simulink model "GaNFET_IMMD_Thermal_Model"  (R2017a)
settings: Solver=VariableStepAuto  StartTime=0.0  StopTime=10.0  RelTol=1e-3
values from neighbouring files (symbols this model uses):
  Rth_jc_FWD2U = 0.12    [Power_loss_calculation.m]
  Rth_jc_IGBT2U = 0.066    [Power_loss_calculation.m]
libraries: fl_lib x29, nesl_utility x2
settings Model: Creator=Caner  LastModifiedBy=Caner

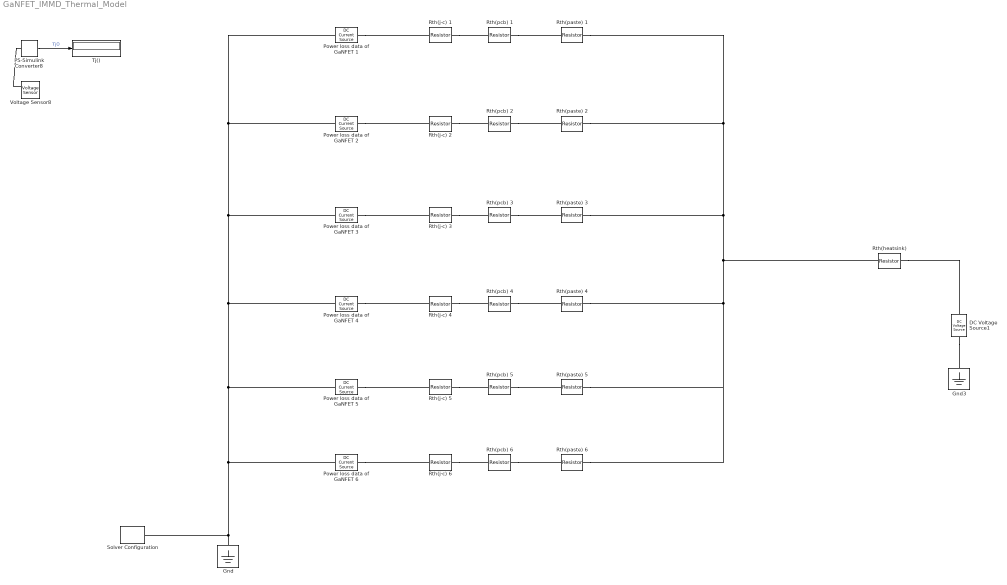
== system GaNFET_IMMD_Thermal_Model ==
  DC Voltage Source1 : fl_lib/Electrical/Electrical Sources/DC Voltage Source  v0=40 V
  Gnd : fl_lib/Electrical/Electrical Elements/Electrical Reference
  Gnd3 : fl_lib/Electrical/Electrical Elements/Electrical Reference
  PS-Simulink Converter8 : nesl_utility/PS-Simulink Converter  PhysicalDomain=network_engine_domain  SubClassName=ps_output  LeftPortType=input  RightPortType=output  PseudoPeriodic=off  Frequencies=[]  Unit=1  AffineConversion=off
  Power loss data of GaNFET 1 : fl_lib/Electrical/Electrical Sources/DC Current Source  i0=PD A
      settings: SourceProductName=Simscape  SourceProductBaseCode=SS
  Power loss data of GaNFET {2..6} (5 alike) : fl_lib/Electrical/Electrical Sources/DC Current Source  i0=PQ A
      settings: SourceProductName=Simscape  SourceProductBaseCode=SS
  "Rth(heatsink) " : fl_lib/Electrical/Electrical Elements/Resistor  R=Rth_jc_IGBT2U Ohm  i_specify=off  i_priority=High  i=0 A  i_nominal_specify=off  i_nominal_unit=A  i_nominal_value=1  v_specify=off  v_priority=High  v=0 V  v_nominal_specify=off  v_nominal_unit=V  v_nominal_value=1
  Rth(j-c) 1 : fl_lib/Electrical/Electrical Elements/Resistor  R=Rth_jc_IGBT2U Ohm  i_specify=off  i_priority=High  i=0 A  i_nominal_specify=off  i_nominal_unit=A  i_nominal_value=1  v_specify=off  v_priority=High  v=0 V  v_nominal_specify=off  v_nominal_unit=V  v_nominal_value=1
  Rth(j-c) {2..6} (5 alike) : fl_lib/Electrical/Electrical Elements/Resistor  R=Rth_jc_FWD2U Ohm  i_specify=off  i_priority=High  i=0 A  i_nominal_specify=off  i_nominal_unit=A  i_nominal_value=1  v_specify=off  v_priority=High  v=0 V  v_nominal_specify=off  v_nominal_unit=V  v_nominal_value=1
  Rth(paste) {1..6} (6 alike) : fl_lib/Electrical/Electrical Elements/Resistor  R=Rth_jc_IGBT2U Ohm  i_specify=off  i_priority=High  i=0 A  i_nominal_specify=off  i_nominal_unit=A  i_nominal_value=1  v_specify=off  v_priority=High  v=0 V  v_nominal_specify=off  v_nominal_unit=V  v_nominal_value=1
  Rth(pcb) {1..6} (6 alike) : fl_lib/Electrical/Electrical Elements/Resistor  R=Rth_jc_IGBT2U Ohm  i_specify=off  i_priority=High  i=0 A  i_nominal_specify=off  i_nominal_unit=A  i_nominal_value=1  v_specify=off  v_priority=High  v=0 V  v_nominal_specify=off  v_nominal_unit=V  v_nominal_value=1
  Solver Configuration : nesl_utility/Solver Configuration  PhysicalDomain=network_engine_domain  SubClassName=solver  LeftPortType=input  RightPortType=generic  Accelerate=off  Tones=[]  Harmonics=[]  SimulateNoise=off  Profile=off  UseLocalSampling=off  EnableSwitchedLinearOptims=on  FrequencyDomain=off  UseCCode=off  RelTol=0.001  AbsTol=1e-06  MinStep=1e-09  ToWorkspace=off  RevertToSquareIcSolve=off  NumHomotopyIterations=100  PhasorMode=off  PhasorModeNumHarmonics=1  OverrideAbsTol=off  DoDC=off  ResidualTolerance=1e-09  UseLocalSolver=off  LocalSolverChoice=NE_BACKWARD_EULER_ADVANCER  LocalSolverSampleTime=0.001  DoFixedCost=off  MaxNonlinIter=3  MaxModeIter=2  LinearAlgebra=Sparse  DelaysMemoryBudget=1024  AutomaticFiltering=on  FilteringTimeConstant=0.001
  Tj() : Display
  Voltage Sensor8 : fl_lib/Electrical/Electrical Sensors/Voltage Sensor
  wires:
  PS-Simulink Converter8/1 -> Tj()/1  "Tj()"
  connections:
  Power loss data of GaNFET 1/LConn1 -- Rth(j-c) 1/LConn1
  Power loss data of GaNFET 2/LConn1 -- Rth(j-c) 2/LConn1
  Gnd/LConn1 -- Power loss data of GaNFET 6/RConn1 -- Power loss data of GaNFET 5/RConn1 -- Power loss data of GaNFET 4/RConn1 -- Power loss data of GaNFET 3/RConn1 -- Power loss data of GaNFET 2/RConn1 -- Power loss data of GaNFET 1/RConn1 -- Solver Configuration/RConn1
  Rth(j-c) 1/RConn1 -- Rth(pcb) 1/LConn1
  Rth(pcb) 1/RConn1 -- Rth(paste) 1/LConn1
  Rth(paste) 1/RConn1 -- Rth(paste) 2/RConn1 -- Rth(paste) 3/RConn1 -- Rth(paste) 6/RConn1 -- Rth(paste) 5/RConn1 -- Rth(paste) 4/RConn1 -- "Rth(heatsink) "/LConn1
  Rth(j-c) 2/RConn1 -- Rth(pcb) 2/LConn1
  Rth(pcb) 2/RConn1 -- Rth(paste) 2/LConn1
  Rth(j-c) 3/RConn1 -- Rth(pcb) 3/LConn1
  Power loss data of GaNFET 3/LConn1 -- Rth(j-c) 3/LConn1
  Rth(pcb) 3/RConn1 -- Rth(paste) 3/LConn1
  Rth(j-c) 4/RConn1 -- Rth(pcb) 4/LConn1
  Power loss data of GaNFET 4/LConn1 -- Rth(j-c) 4/LConn1
  Rth(pcb) 4/RConn1 -- Rth(paste) 4/LConn1
  Rth(j-c) 5/RConn1 -- Rth(pcb) 5/LConn1
  Power loss data of GaNFET 5/LConn1 -- Rth(j-c) 5/LConn1
  Rth(pcb) 5/RConn1 -- Rth(paste) 5/LConn1
  Rth(j-c) 6/RConn1 -- Rth(pcb) 6/LConn1
  Power loss data of GaNFET 6/LConn1 -- Rth(j-c) 6/LConn1
  Rth(pcb) 6/RConn1 -- Rth(paste) 6/LConn1
  DC Voltage Source1/RConn1 -- Gnd3/LConn1
  "Rth(heatsink) "/RConn1 -- DC Voltage Source1/LConn1
  Voltage Sensor8/RConn1 -- PS-Simulink Converter8/LConn1
